simulink library "aero_sim_lib"  (Simulink 7.1)
undefined symbols (not defined in the file or in its folder): DiscIntNeverNeededParam, M, T0, tau_motor, ToverTh, Vb0, W0, X0
libraries: aero_sim_lib x24, simulink x16
(part 1 of 2)
settings Model: Creator=Administrator  LastModifiedBy=nkottens

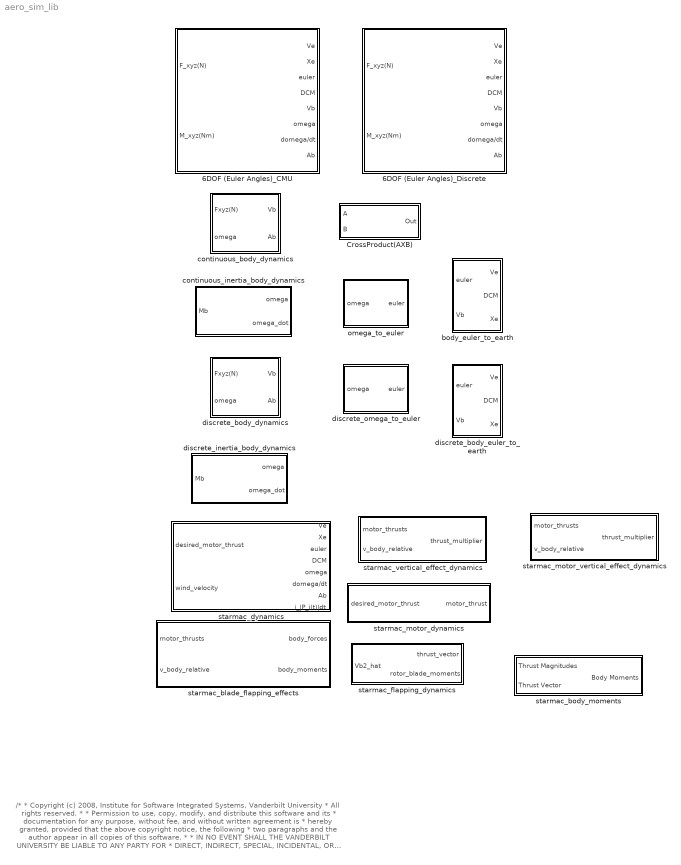
== system aero_sim_lib ==
  note: /*
      |  * Copyright (c) 2008, Institute for Software Integrated Systems, Vanderbilt University
      |  * All rights reserved.
      |  *
      |  * Permission to use, copy, modify, and distribute this software and its
      |  * documentation for any purpose, without fee, and without written agreement is
      |  * hereby granted, provided that the above copyright notice, the following
      |  * two paragraphs and the author appear in all copies of this software.
      |  *
      |  * IN NO EVENT SHALL THE VANDERBILT UNIVERSITY BE LIABLE TO ANY PARTY FOR
      |  * DIRECT, INDIRECT, SPECIAL, INCIDENTAL, OR CONSEQUENTIAL DAMAGES ARISING OUT
      |  * OF THE USE OF THIS SOFTWARE AND ITS DOCUMENTATION, EVEN IF THE VANDERBILT
      |  * UNIVERSITY HAS BEEN ADVISED OF THE POSSIBILITY OF SUCH DAMAGE.
      |  *
      |  * THE VANDERBILT UNIVERSITY SPECIFICALLY DISCLAIMS ANY WARRANTIES,
      |  * INCLUDING, BUT NOT LIMITED TO, THE IMPLIED WARRANTIES OF MERCHANTABILITY
      |  * AND FITNESS FOR A PARTICULAR PURPOSE.  THE SOFTWARE PROVIDED HEREUNDER IS
      |  * ON AN "AS IS" BASIS, AND THE VANDERBILT UNIVERSITY HAS NO OBLIGATION TO
      |  * PROVIDE MAINTENANCE, SUPPORT, UPDATES, ENHANCEMENTS, OR MODIFICATIONS.
      |  *
      |  * @author Nicholas Kottenstette
      |  */
  6DOF (Euler Angles)_CMU : Subsystem  mask{XYZe_0=zeros(3,1), Vb_0=zeros(3,1), euler_0=zeros(3,1), omega_0=zeros(3,1), M=1, I=eye(3)}
      mask prompts: XYZe_0 "Initial position in inertial axes [Xe,Ye,Ze]:"; Vb_0 "Initial velocity in body axes [U,v,w]:"; euler_0 "Initial Euler orientation [roll, pitch, yaw]=[phi,theta,psi]:"; omega_0 "Initial body rotation rates [p,q,r]=omega:"; M "Initial mass:"; I "Inertial:"
  6DOF (Euler Angles)_Discrete : Subsystem  AncestorBlock=aero_sim_lib/6DOF (Euler Angles)_CMU  mask{XYZe_0=zeros(3,1), Vb_0=zeros(3,1), euler_0=zeros(3,1), omega_0=zeros(3,1), M=1, I=eye(3), T_int=1.0}
      mask prompts: XYZe_0 "Initial position in inertial axes [Xe,Ye,Ze]:"; Vb_0 "Initial velocity in body axes [U,v,w]:"; euler_0 "Initial Euler orientation [roll, pitch, yaw]=[phi,theta,psi]:"; omega_0 "Initial body rotation rates [p,q,r]=omega:"; M "Initial mass:"; I "Inertial:"; T_int "Integrator Period:"
  CrossProduct(AXB) : Subsystem
      mask Description: Out = A x B
  body_euler_to_earth : Subsystem  AncestorBlock=aero_sim_lib/6DOF (Euler Angles)_CMU/body_euler_to_earth  mask{XYZe_0=zeros(3,1)}
      mask prompts: XYZe_0 "Initial position in inertial axes [Xe,Ye,Ze]:"
  continuous_body_dynamics : Subsystem  AncestorBlock=aero_sim_lib/6DOF (Euler Angles)_CMU/continuous_body_dynamics  mask{M=1, Vb_0=zeros(3,1)}
      mask prompts: M "Initial Mass:"; Vb_0 "Initial velocity in body axes [u,v,w]:"
  continuous_inertia_body_dynamics : Subsystem  AncestorBlock=aero_sim_lib/6DOF (Euler Angles)_CMU/continuous_inertia_body_dynamics  mask{I=eye(3), omega_0=zeros(3,1)}
      mask prompts: I "Inertia:"; omega_0 "Initial body rotation rates [p,q,r]=omega:"
  discrete_body_dynamics : Subsystem  AncestorBlock=aero_sim_lib/continuous_body_dynamics  mask{M=1, Vb_0=zeros(3,1), T_int=1.0}
      mask prompts: M "Initial Mass:"; Vb_0 "Initial velocity in body axes [u,v,w]:"; T_int "Integrator Period"
  discrete_body_euler_to_earth : Subsystem  AncestorBlock=aero_sim_lib/body_euler_to_earth  mask{XYZe_0=zeros(3,1), T_int=1.0}
      mask prompts: XYZe_0 "Initial position in inertial axes [Xe,Ye,Ze]:"; T_int "Integrator Period:"
  discrete_inertia_body_dynamics : Subsystem  AncestorBlock=aero_sim_lib/continuous_inertia_body_dynamics  mask{I=eye(3), omega_0=zeros(3,1), T_int=1.0}
      mask prompts: I "Inertia:"; omega_0 "Initial body rotation rates [p,q,r]=omega:"; T_int "Integrator Period:"
  discrete_omega_to_euler : Subsystem  AncestorBlock=aero_sim_lib/omega_to_euler  mask{euler_0=zeros(3,1), T_int=1.0}
      mask prompts: euler_0 "Initial Euler orientation [roll,pitch,yaw]:"; T_int "Integrator Period:"
  omega_to_euler : Subsystem  AncestorBlock=aero_sim_lib/6DOF (Euler Angles)_CMU/omega_to_euler  mask{euler_0=zeros(3,1)}
      mask prompts: euler_0 "Initial Euler orientation [roll,pitch,yaw]:"
  starmac_blade_flapping_effects : Subsystem  AncestorBlock=aero_sim_lib/starmac_dynamics/starmac_blade_flapping_effects
  starmac_body_moments : Subsystem  mask{dx=.3048, dz=.07, K_torque=.47}
  starmac_dynamics : Subsystem
  starmac_flapping_dynamics : Subsystem  mask{K_a1s=.009, K_beta=.23}
  starmac_motor_dynamics : Subsystem  AncestorBlock=aero_sim_lib/starmac_dynamics/starmac_motor_dynamics  mask{tau_motor=tau_motor, T_nom=M*9.8/4, thrust_max=9.8, thrust_min=0, motor_lag_enable=on, motor_variance=.01*(.05*9.8/4)^2, Ts=1/76}
      mask prompts: tau_motor "tau_motor (seconds):"; T_nom "nominal thrust (N):"; thrust_max "maximum thrust (N):"; thrust_min "minimum thrust (N):"; motor_lag_enable "Motor Lag Enabled:"; motor_variance "Motor Variance [motor_variance]:"; Ts "Motor Update Rate (seconds):"
  starmac_motor_vertical_effect_dynamics : Subsystem  mask{tau_motor=tau_motor, R=0.127, Alpha=(pi/180)*[-85:5:85], Vinf=[0:0.5:6], Vh=sqrt(9.8*[0.3:0.02:0.8]/(2*1.2*pi*.127^2)), ToverTh=ones(35,13,26)}
      mask prompts: tau_motor "motor time constant (s)"; R "radius of propeller (m)"; Alpha "Alpha (radians):"; Vinf "Vinf (m/s):"; Vh "Vh (m/s):"
      mask init:
      | rho=1.2;    % kg/m^3, density of air
      | A = pi*R^2; % m^2, area swept out by 1 rotor
  starmac_vertical_effect_dynamics : Subsystem  mask{tau_motor=tau_motor, R=0.127, Alpha=(pi/180)*[-85:5:85], Vinf=[0:0.5:6], Thrust=9.8*[0.3:0.02:0.8]}
      mask prompts: tau_motor "motor time constant (s)"; R "radius of propeller (m)"; Alpha "Alpha (radians)"; Vinf "Vinf (radians)"; Thrust "Propeller Thrust (N)"
      mask init:
      | rho = 1.2;
      | A = pi*R^2;
      | Vh = sqrt(Thrust/(2*rho*A));
      | for i = 1:length(Vh)
      |     for j = 1:length(Vinf)
      |         for k = 1:length(Alpha)
      |             Vi(k,j,i) = find_vi(Vh(i),Vinf(j),Alpha(k));
      |             ToverTh(k,j,i) = min(10,max(0.1,Vh(i)/(Vi(k,j,i)+Vinf(j)*sin(Alpha(k)))));
      |         end
      |     end
      | end

== system aero_sim_lib/6DOF (Euler Angles)_CMU ==
  note: 6 DOF System Model
  note: This subsystem models a 6 degree of freedom (6DOF) system in Euler angles.
      | A Direct Cosine Matrix (DCM) is produced to allow for easy transformations to
      | and from the reference frame of the body.  Enter appropriate Parameters in the dialog menu.
      | Follows Euler Angle Sequence (1,2,3), see Section 5.6, Representing Attitude: Euler Angles, Unit
      | Quaternions, and Rotation by James Diebel.  Interface matches that from the Aerospace Toolbox
      | for non variable mass (6DoF EoM (Body Axis) for Euler Angles).
      |
      | J. Kapinski
      | Carnegia Mellon University
      | 7/2007
      | Revised:
      | Nicholas Kottenstette, ISIS, 8/2008
  F_xyz(N) : Inport  OutDataType=sfix(16)  OutScaling=2^0
  M_xyz(Nm) : Inport  Port=2  PortDimensions=3  OutDataType=sfix(16)  OutScaling=2^0
  body_euler_to_earth : aero_sim_lib/body_euler_to_earth  SystemSampleTime=-1  XYZe_0=XYZe_0
  continuous_body_dynamics : aero_sim_lib/continuous_body_dynamics  SystemSampleTime=-1  M=M  Vb_0=Vb_0
  continuous_inertia_body_dynamics : aero_sim_lib/continuous_inertia_body_dynamics  SystemSampleTime=-1  I=I  omega_0=omega_0
  omega_to_euler : aero_sim_lib/omega_to_euler  SystemSampleTime=-1  euler_0=euler_0
  Ve : Outport  OutDataType=sfix(16)  OutScaling=2^0
  Xe : Outport  Port=2  OutDataType=sfix(16)  OutScaling=2^0
  euler : Outport  Port=3  OutDataType=sfix(16)  OutScaling=2^0
  DCM : Outport  Port=4  OutDataType=sfix(16)  OutScaling=2^0
  Vb : Outport  Port=5  OutDataType=sfix(16)  OutScaling=2^0
  omega : Outport  Port=6  OutDataType=sfix(16)  OutScaling=2^0
  domega/dt : Outport  Port=7  OutDataType=sfix(16)  OutScaling=2^0
  Ab : Outport  Port=8  OutDataType=sfix(16)  OutScaling=2^0
  wires:
  M_xyz(Nm)/1 -> continuous_inertia_body_dynamics/1
  F_xyz(N)/1 -> continuous_body_dynamics/1
  continuous_inertia_body_dynamics/1 -> omega/1, continuous_body_dynamics/2, omega_to_euler/1
  continuous_body_dynamics/1 -> Vb/1, body_euler_to_earth/2
  continuous_body_dynamics/2 -> Ab/1
  continuous_inertia_body_dynamics/2 -> domega/dt/1
  omega_to_euler/1 -> euler/1, body_euler_to_earth/1
  body_euler_to_earth/1 -> Ve/1
  body_euler_to_earth/2 -> DCM/1
  body_euler_to_earth/3 -> Xe/1

== system aero_sim_lib/6DOF (Euler Angles)_Discrete ==
  note: This subsystem models a 6 degree of freedom (6DOF) system in Euler angles.
      | A Direct Cosine Matrix (DCM) is produced to allow for easy transformations to
      | and from the reference frame of the body.  Enter appropriate Parameters in the dialog menu.
      | Follows Euler Angle Sequence (1,2,3), see Section 5.6, Representing Attitude: Euler Angles, Unit
      | Quaternions, and Rotation by James Diebel.  Interface matches that from the Aerospace Toolbox
      | for non variable mass (6DoF EoM (Body Axis) for Euler Angles).
      |
      | J. Kapinski
      | Carnegia Mellon University
      | 7/2007
      | Revised:
      | Nicholas Kottenstette, ISIS, 8/2008
  note: 6 DOF System Model
  F_xyz(N) : Inport
  M_xyz(Nm) : Inport  Port=2  PortDimensions=3
  discrete_body_dynamics : aero_sim_lib/discrete_body_dynamics  SystemSampleTime=-1  M=M  Vb_0=Vb_0  T_int=T_int
  discrete_body_euler_to_earth : aero_sim_lib/discrete_body_euler_to_earth  SystemSampleTime=-1  XYZe_0=XYZe_0  T_int=T_int
  discrete_inertia_body_dynamics : aero_sim_lib/discrete_inertia_body_dynamics  SystemSampleTime=-1  I=I  omega_0=omega_0  T_int=T_int
  discrete_omega_to_euler : aero_sim_lib/discrete_omega_to_euler  SystemSampleTime=-1  euler_0=euler_0  T_int=T_int
  Ve : Outport
  Xe : Outport  Port=2
  euler : Outport  Port=3
  DCM : Outport  Port=4
  Vb : Outport  Port=5
  omega : Outport  Port=6
  domega/dt : Outport  Port=7
  Ab : Outport  Port=8
  wires:
  discrete_body_dynamics/2 -> Ab/1
  discrete_body_dynamics/1 -> Vb/1, discrete_body_euler_to_earth/2
  F_xyz(N)/1 -> discrete_body_dynamics/1
  discrete_omega_to_euler/1 -> euler/1, discrete_body_euler_to_earth/1
  discrete_body_euler_to_earth/1 -> Ve/1
  discrete_body_euler_to_earth/2 -> DCM/1
  discrete_body_euler_to_earth/3 -> Xe/1
  M_xyz(Nm)/1 -> discrete_inertia_body_dynamics/1
  discrete_inertia_body_dynamics/1 -> omega/1, discrete_omega_to_euler/1, discrete_body_dynamics/2
  discrete_inertia_body_dynamics/2 -> domega/dt/1

== system aero_sim_lib/CrossProduct(AXB) ==
  A : Inport  OutDataType=sfix(16)  OutScaling=2^0
  B : Inport  Port=2  OutDataType=sfix(16)  OutScaling=2^0
  Fcn : Fcn  Expr=u[2]*u[6]-u[3]*u[5]
  Fcn1 : Fcn  Expr=u[3]*u[4]-u[1]*u[6]
  Fcn2 : Fcn  Expr=u[1]*u[5]-u[2]*u[4]
  Mux : Mux  Inputs=2
  Mux1 : Mux  Inputs=3
  Out : Outport  OutDataType=sfix(16)  OutScaling=2^0
  wires:
  Mux1/1 -> Out/1
  Fcn2/1 -> Mux1/3
  Fcn1/1 -> Mux1/2
  Fcn/1 -> Mux1/1
  Mux/1 -> Fcn2/1, Fcn1/1, Fcn/1
  B/1 -> Mux/2
  A/1 -> Mux/1

== system aero_sim_lib/body_euler_to_earth ==
  euler : Inport  OutDataType=sfix(16)  OutScaling=2^0
  Vb : Inport  Port=2  OutDataType=sfix(16)  OutScaling=2^0
  Constant : Constant  Value=XYZe_0  OutDataType=sfix(16)  OutScaling=2^0
  Create_DCM : Subsystem
  Math Function : Math  Operator=transpose  OutDataType=sfix(16)  OutScaling=2^0  SaturateOnIntegerOverflow=on
  Position : Integrator  InitialConditionSource=external  InitialCondition=X0
  Product2 : Product  Multiplication=Matrix(*)  OutDataType=sfix(16)  OutScaling=2^0  RndMeth=Zero
  Ve : Outport  OutDataType=sfix(16)  OutScaling=2^0
  DCM : Outport  Port=2  OutDataType=sfix(16)  OutScaling=2^0
  Xe : Outport  Port=3  OutDataType=sfix(16)  OutScaling=2^0
  wires:
  Vb/1 -> Product2/2
  euler/1 -> Create_DCM/1(euler)
  Create_DCM/1(DCM) -> Math Function/1, DCM/1
  Math Function/1 -> Product2/1
  Product2/1 -> Position/1, Ve/1
  Position/1 -> Xe/1
  Constant/1 -> Position/2

== system aero_sim_lib/continuous_body_dynamics ==
  note: Vb_dot
  Fxyz(N) : Inport  OutDataType=sfix(16)  OutScaling=2^0
  omega : Inport  Orientation=down  Port=2  OutDataType=sfix(16)  OutScaling=2^0
  Constant : Constant  Value=Vb_0  OutDataType=sfix(16)  OutScaling=2^0
  CrossProduct(AXB) : aero_sim_lib/CrossProduct(AXB)  Orientation=left  SystemSampleTime=-1
  Gain : Gain  Gain=1/M  ParameterDataType=sfix(16)  ParameterScaling=2^0  OutDataType=sfix(16)  OutScaling=2^0
  Sum : Sum  Inputs=|+-  OutDataType=sfix(16)  OutScaling=2^0
  Velocity : Integrator  InitialConditionSource=external  InitialCondition=Vb0
  Vb : Outport  OutDataType=sfix(16)  OutScaling=2^0
  Ab : Outport  Port=2  OutDataType=sfix(16)  OutScaling=2^0
  wires:
  Constant/1 -> Velocity/2
  Fxyz(N)/1 -> Gain/1
  omega/1 -> CrossProduct(AXB)/1
  Gain/1 -> Ab/1, Sum/1
  CrossProduct(AXB)/1 -> Sum/2
  Sum/1 -> Velocity/1
  Velocity/1 -> Vb/1, CrossProduct(AXB)/2  "V"

== system aero_sim_lib/continuous_inertia_body_dynamics ==
  Mb : Inport  OutDataType=sfix(16)  OutScaling=2^0
  Constant : Constant  Value=inv(I)  OutDataType=sfix(16)  OutScaling=2^0
  Constant1 : Constant  Value=I  OutDataType=sfix(16)  OutScaling=2^0
  Constant2 : Constant  Value=omega_0  OutDataType=sfix(16)  OutScaling=2^0
  CrossProduct(AXB) : aero_sim_lib/CrossProduct(AXB)  SystemSampleTime=-1
  Product : Product  Multiplication=Matrix(*)  OutDataType=sfix(16)  OutScaling=2^0  RndMeth=Zero
  Product1 : Product  Multiplication=Matrix(*)  OutDataType=sfix(16)  OutScaling=2^0  RndMeth=Zero
  Sum1 : Sum  Inputs=|-+  OutDataType=sfix(16)  OutScaling=2^0
  integrator : Integrator  InitialConditionSource=external  InitialCondition=W0
  omega : Outport  OutDataType=sfix(16)  OutScaling=2^0
  omega_dot : Outport  Port=2  OutDataType=sfix(16)  OutScaling=2^0
  wires:
  Product1/1 -> CrossProduct(AXB)/2
  Constant1/1 -> Product1/1
  Mb/1 -> Sum1/2
  CrossProduct(AXB)/1 -> Sum1/1
  integrator/1 -> Product1/2, CrossProduct(AXB)/1, omega/1
  Sum1/1 -> Product/2
  Constant2/1 -> integrator/2
  Constant/1 -> Product/1
  Product/1 -> omega_dot/1, integrator/1

== system aero_sim_lib/discrete_body_dynamics ==
  note: Vb_dot
  Fxyz(N) : Inport
  omega : Inport  Orientation=down  Port=2
  Constant : Constant  Value=Vb_0
  CrossProduct(AXB) : aero_sim_lib/CrossProduct(AXB)  Orientation=left  SystemSampleTime=-1
  Discrete-Time Integrator : DiscreteIntegrator  IntegratorMethod=Integration: Trapezoidal  InitialConditionSource=external  SampleTime=T_int  ICPrevOutput=DiscIntNeverNeededParam  ICPrevScaledInput=DiscIntNeverNeededParam
  Gain : Gain  Gain=1/M
  Sum : Sum  Inputs=|+-
  Vb : Outport
  Ab : Outport  Port=2
  wires:
  Discrete-Time Integrator/1 -> CrossProduct(AXB)/2, Vb/1  "V"
  Sum/1 -> Discrete-Time Integrator/1
  CrossProduct(AXB)/1 -> Sum/2
  Gain/1 -> Sum/1, Ab/1
  omega/1 -> CrossProduct(AXB)/1
  Fxyz(N)/1 -> Gain/1
  Constant/1 -> Discrete-Time Integrator/2

== system aero_sim_lib/discrete_body_euler_to_earth ==
  euler : Inport
  Vb : Inport  Port=2
  Constant : Constant  Value=XYZe_0
  Create_DCM : Subsystem
  Discrete-Time Integrator : DiscreteIntegrator  IntegratorMethod=Integration: Trapezoidal  InitialConditionSource=external  SampleTime=T_int  ICPrevOutput=DiscIntNeverNeededParam  ICPrevScaledInput=DiscIntNeverNeededParam
  Math Function : Math  Operator=transpose  SaturateOnIntegerOverflow=on
  Product2 : Product  Multiplication=Matrix(*)  RndMeth=Zero
  Ve : Outport
  DCM : Outport  Port=2
  Xe : Outport  Port=3
  wires:
  Constant/1 -> Discrete-Time Integrator/2
  Discrete-Time Integrator/1 -> Xe/1
  Product2/1 -> Ve/1, Discrete-Time Integrator/1
  Math Function/1 -> Product2/1
  Create_DCM/1(DCM) -> DCM/1, Math Function/1
  euler/1 -> Create_DCM/1(euler)
  Vb/1 -> Product2/2

== system aero_sim_lib/discrete_inertia_body_dynamics ==
  Mb : Inport
  Constant : Constant  Value=inv(I)
  Constant1 : Constant  Value=I
  Constant2 : Constant  Value=omega_0
  CrossProduct(AXB) : aero_sim_lib/CrossProduct(AXB)  SystemSampleTime=-1
  Discrete-Time Integrator : DiscreteIntegrator  IntegratorMethod=Integration: Trapezoidal  InitialConditionSource=external  SampleTime=T_int  ICPrevOutput=DiscIntNeverNeededParam  ICPrevScaledInput=DiscIntNeverNeededParam
  Product : Product  Multiplication=Matrix(*)  RndMeth=Zero
  Product1 : Product  Multiplication=Matrix(*)  RndMeth=Zero
  Sum1 : Sum  Inputs=|-+
  omega : Outport
  omega_dot : Outport  Port=2
  wires:
  Product/1 -> omega_dot/1, Discrete-Time Integrator/1
  Constant/1 -> Product/1
  Constant2/1 -> Discrete-Time Integrator/2
  Sum1/1 -> Product/2
  Discrete-Time Integrator/1 -> omega/1, CrossProduct(AXB)/1, Product1/2
  CrossProduct(AXB)/1 -> Sum1/1
  Mb/1 -> Sum1/2
  Constant1/1 -> Product1/1
  Product1/1 -> CrossProduct(AXB)/2

== system aero_sim_lib/discrete_omega_to_euler ==
  omega : Inport  PortDimensions=3
  Body-based-to-ref-frame-based : Subsystem
  Constant : Constant  Value=euler_0
  Discrete-Time Integrator : DiscreteIntegrator  IntegratorMethod=Integration: Trapezoidal  InitialConditionSource=external  SampleTime=T_int  ICPrevOutput=DiscIntNeverNeededParam  ICPrevScaledInput=DiscIntNeverNeededParam
  euler : Outport
  wires:
  Body-based-to-ref-frame-based/1(deuler/dt) -> Discrete-Time Integrator/1
  Discrete-Time Integrator/1 -> Body-based-to-ref-frame-based/2(euler), euler/1
  Constant/1 -> Discrete-Time Integrator/2
  omega/1 -> Body-based-to-ref-frame-based/1(omega)

== system aero_sim_lib/omega_to_euler ==
  omega : Inport  PortDimensions=3  OutDataType=sfix(16)  OutScaling=2^0
  Body-based-to-ref-frame-based : Subsystem
  Constant : Constant  Value=euler_0  OutDataType=sfix(16)  OutScaling=2^0
  integrator : Integrator  InitialConditionSource=external  InitialCondition=T0
  euler : Outport  OutDataType=sfix(16)  OutScaling=2^0
  wires:
  omega/1 -> Body-based-to-ref-frame-based/1(omega)
  Constant/1 -> integrator/2
  integrator/1 -> euler/1, Body-based-to-ref-frame-based/2(euler)
  Body-based-to-ref-frame-based/1(deuler/dt) -> integrator/1

== system aero_sim_lib/starmac_blade_flapping_effects ==
  motor_thrusts : Inport  OutDataType=sfix(16)  OutScaling=2^0
  v_body_relative : Inport  Port=2  OutDataType=sfix(16)  OutScaling=2^0
  Pick First 2 Elements : Constant  Value=[1 0 0; 0 1 0; 0 0 0]  OutDataType=sfix(16)  OutScaling=2^0
  Product : Product  OutDataType=sfix(16)  OutScaling=2^0  RndMeth=Zero
  Product2 : Product  Multiplication=Matrix(*)  OutDataType=sfix(16)  OutScaling=2^0  RndMeth=Zero
  Product4 : Product  OutDataType=sfix(16)  OutScaling=2^0  RndMeth=Zero
  Sum : Sum  Inputs=|++  OutDataType=sfix(16)  OutScaling=2^0
  Sum of Elements : Sum  Inputs=+  OutDataType=sfix(16)  OutScaling=2^-10
  starmac_body_moments : Subsystem  AncestorBlock=aero_sim_lib/starmac_body_moments  mask{dx=.3048, dz=.07, K_torque=.47}
  starmac_flapping_dynamics : Subsystem  AncestorBlock=aero_sim_lib/starmac_flapping_dynamics  mask{K_a1s=.009, K_beta=.23}
  starmac_vertical_effect_dynamics : Subsystem  AncestorBlock=aero_sim_lib/starmac_vertical_effect_dynamics  mask{tau_motor=0.1, R=0.127, Alpha=(pi/180)*[-85:5:85], Vinf=[0:0.5:6], Thrust=9.8*[0.3:0.02:0.8]}
      mask prompts: tau_motor "motor time constant (s)"; R "radius of propeller (m)"; Alpha "Alpha (radians)"; Vinf "Vinf (radians)"; Thrust "Propeller Thrust (N)"
      mask init: same as aero_sim_lib/starmac_vertical_effect_dynamics
  body_forces : Outport  OutDataType=sfix(16)  OutScaling=2^0
  body_moments : Outport  Port=2  OutDataType=sfix(16)  OutScaling=2^0
  wires:
  Product/1 -> starmac_body_moments/1(Thrust Magnitudes), Sum of Elements/1
  starmac_vertical_effect_dynamics/1(thrust_multiplier) -> Product/2
  motor_thrusts/1 -> starmac_vertical_effect_dynamics/1(motor_thrusts), Product/1
  Pick First 2 Elements/1 -> Product2/1
  v_body_relative/1 -> starmac_vertical_effect_dynamics/2(v_body_relative), Product2/2
  Product2/1 -> starmac_flapping_dynamics/1(Vb2_hat)
  Sum of Elements/1 -> Product4/1
  Product4/1 -> body_forces/1
  starmac_flapping_dynamics/1(thrust_vector) -> starmac_body_moments/2(Thrust Vector), Product4/2
  starmac_body_moments/1(Body Moments) -> Sum/1
  Sum/1 -> body_moments/1
  starmac_flapping_dynamics/2(rotor_blade_moments) -> Sum/2

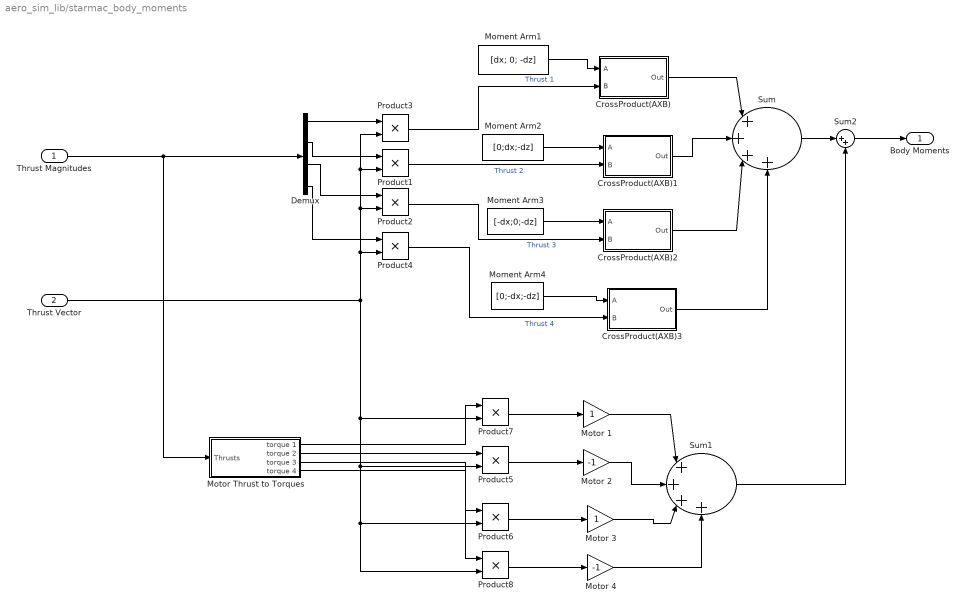
== system aero_sim_lib/starmac_body_moments ==
  Thrust Magnitudes : Inport  OutDataType=sfix(16)  OutScaling=2^0
  Thrust Vector : Inport  Port=2  OutDataType=sfix(16)  OutScaling=2^0
  CrossProduct(AXB) : Subsystem
  CrossProduct(AXB)1 : Subsystem
  CrossProduct(AXB)2 : Subsystem
  CrossProduct(AXB)3 : Subsystem
  Demux : Demux
  Moment Arm1 : Constant  Value=[dx; 0; -dz]  OutDataType=sfix(16)  OutScaling=2^0
  Moment Arm2 : Constant  Value=[0;dx;-dz]  OutDataType=sfix(16)  OutScaling=2^0
  Moment Arm3 : Constant  Value=[-dx;0;-dz]  OutDataType=sfix(16)  OutScaling=2^0
  Moment Arm4 : Constant  Value=[0;-dx;-dz]  OutDataType=sfix(16)  OutScaling=2^0
  Motor 1 : Gain  ParameterDataType=sfix(16)  ParameterScaling=2^0  OutDataType=sfix(16)  OutScaling=2^0
  Motor 2 : Gain  Gain=-1  ParameterDataType=sfix(16)  ParameterScaling=2^0  OutDataType=sfix(16)  OutScaling=2^0
  Motor 3 : Gain  ParameterDataType=sfix(16)  ParameterScaling=2^0  OutDataType=sfix(16)  OutScaling=2^0
  Motor 4 : Gain  Gain=-1  ParameterDataType=sfix(16)  ParameterScaling=2^0  OutDataType=sfix(16)  OutScaling=2^0
  Motor Thrust to Torques : Subsystem
  Product{1..8} (8 alike) : Product  OutDataType=sfix(16)  OutScaling=2^0  RndMeth=Zero
  Sum : Sum  Inputs=|++++  OutDataType=sfix(16)  OutScaling=2^0
  Sum1 : Sum  Inputs=|++++  OutDataType=sfix(16)  OutScaling=2^0
  Sum2 : Sum  Inputs=|++  OutDataType=sfix(16)  OutScaling=2^0
  Body Moments : Outport  OutDataType=sfix(16)  OutScaling=2^0
  wires:
  CrossProduct(AXB)1/1(Out) -> Sum/2
  Motor Thrust to Torques/4(torque 4) -> Product8/1
  Motor Thrust to Torques/3(torque 3) -> Product6/1
  Motor Thrust to Torques/2(torque 2) -> Product5/1
  Motor Thrust to Torques/1(torque 1) -> Product7/1
  Product8/1 -> Motor 4/1
  Product6/1 -> Motor 3/1
  Product5/1 -> Motor 2/1
  Product7/1 -> Motor 1/1
  Sum2/1 -> Body Moments/1
  Sum1/1 -> Sum2/2
  Sum/1 -> Sum2/1
  Motor 4/1 -> Sum1/4
  Motor 3/1 -> Sum1/3
  Motor 2/1 -> Sum1/2
  Motor 1/1 -> Sum1/1
  CrossProduct(AXB)3/1(Out) -> Sum/4
  CrossProduct(AXB)2/1(Out) -> Sum/3
  CrossProduct(AXB)/1(Out) -> Sum/1
  Product4/1 -> CrossProduct(AXB)3/2(B)  "Thrust 4"
  Moment Arm4/1 -> CrossProduct(AXB)3/1(A)
  Product2/1 -> CrossProduct(AXB)2/2(B)  "Thrust 3"
  Moment Arm3/1 -> CrossProduct(AXB)2/1(A)
  Product1/1 -> CrossProduct(AXB)1/2(B)  "Thrust 2"
  Moment Arm2/1 -> CrossProduct(AXB)1/1(A)
  Product3/1 -> CrossProduct(AXB)/2(B)  "Thrust 1"
  Moment Arm1/1 -> CrossProduct(AXB)/1(A)
  Thrust Vector/1 -> Product8/2, Product6/2, Product5/2, Product7/2, Product4/2, Product2/2, Product1/2, Product3/2
  Demux/4 -> Product4/1
  Demux/3 -> Product2/1
  Demux/2 -> Product1/1
  Demux/1 -> Product3/1
  Thrust Magnitudes/1 -> Motor Thrust to Torques/1(Thrusts), Demux/1

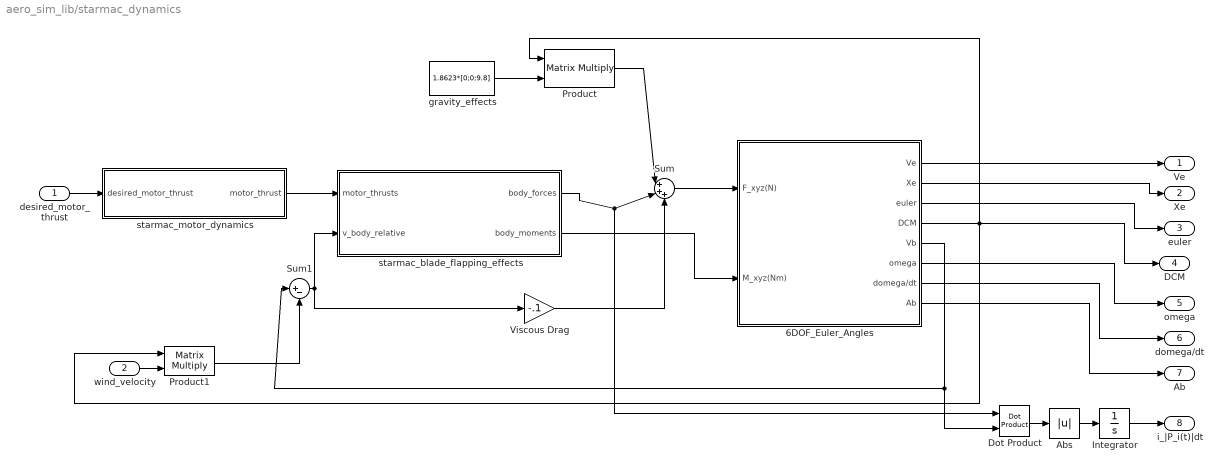
== system aero_sim_lib/starmac_dynamics ==
  desired_motor_thrust : Inport  OutDataType=sfix(16)  OutScaling=2^0
  wind_velocity : Inport  Port=2  OutDataType=sfix(16)  OutScaling=2^0
  6DOF_Euler_Angles : Subsystem  AncestorBlock=aero_sim_lib/6DOF (Euler Angles)_CMU  mask{XYZe_0=[0.1;0.2;0], Vb_0=[0;0;0], euler_0=[0;0;0], omega_0=[0;0;0], M=1.8623, I=diag([0.02759 0.02771 0.04806])}
      mask prompts: XYZe_0 "Initial position in inertial axes [Xe,Ye,Ze]:"; Vb_0 "Initial velocity in body axes [U,v,w]:"; euler_0 "Initial Euler orientation [roll, pitch, yaw]=[phi,theta,psi]:"; omega_0 "Initial body rotation rates [p,q,r]=omega:"; M "Initial mass:"; I "Inertial:"
  Abs : Abs  OutDataType=sfix(16)  OutScaling=2^0
  Dot Product : simulink/Math Operations/Dot Product  InputSameDT=on  OutDataType=sfix(16)  OutScaling=2^-10  DoSatur=off
  Integrator : Integrator
  Product : Product  Multiplication=Matrix(*)  OutDataType=sfix(16)  OutScaling=2^0  RndMeth=Zero
  Product1 : Product  Multiplication=Matrix(*)  OutDataType=sfix(16)  OutScaling=2^0  RndMeth=Zero
  Sum : Sum  Inputs=|+++  OutDataType=sfix(16)  OutScaling=2^0
  Sum1 : Sum  Inputs=|+-  OutDataType=sfix(16)  OutScaling=2^0
  Viscous Drag : Gain  Gain=-.1  ParameterDataType=sfix(16)  ParameterScaling=2^0  OutDataType=sfix(16)  OutScaling=2^0
  gravity_effects : Constant  Value=1.8623*[0;0;9.8]  OutDataType=sfix(16)  OutScaling=2^0
  starmac_blade_flapping_effects : Subsystem  AncestorBlock=aero_sim_lib/starmac_blade_flapping_effects
  starmac_motor_dynamics : Subsystem  AncestorBlock=aero_sim_lib/starmac_motor_dynamics  mask{tau_motor=.1, T_nom=1.8263*9.8/4, thrust_max=9.8, thrust_min=0, motor_lag_enable=on, motor_variance=.01*(.05*9.8/4)^2, Ts=1/76}
      mask prompts: tau_motor "tau_motor (seconds):"; T_nom "nominal thrust (N):"; thrust_max "maximum thrust (N):"; thrust_min "minimum thrust (N):"; motor_lag_enable "Motor Lag Enabled:"; motor_variance "Motor Variance [motor_variance]:"; Ts "Motor Update Rate (seconds):"
  Ve : Outport  OutDataType=sfix(16)  OutScaling=2^0
  Xe : Outport  Port=2  OutDataType=sfix(16)  OutScaling=2^0
  euler : Outport  Port=3  OutDataType=sfix(16)  OutScaling=2^0
  DCM : Outport  Port=4  OutDataType=sfix(16)  OutScaling=2^0
  omega : Outport  Port=5  OutDataType=sfix(16)  OutScaling=2^0
  domega/dt : Outport  Port=6  OutDataType=sfix(16)  OutScaling=2^0
  Ab : Outport  Port=7  OutDataType=sfix(16)  OutScaling=2^0
  i_|P_i(t)|dt : Outport  Port=8  OutDataType=sfix(16)  OutScaling=2^0
  wires:
  wind_velocity/1 -> Product1/2
  desired_motor_thrust/1 -> starmac_motor_dynamics/1(desired_motor_thrust)
  starmac_blade_flapping_effects/1(body_forces) -> Sum/2, Dot Product/1
  starmac_blade_flapping_effects/2(body_moments) -> 6DOF_Euler_Angles/2(M_xyz(Nm))
  Viscous Drag/1 -> Sum/3
  6DOF_Euler_Angles/5(Vb) -> Sum1/1, Dot Product/2
  Product1/1 -> Sum1/2
  Sum1/1 -> Viscous Drag/1, starmac_blade_flapping_effects/2(v_body_relative)
  gravity_effects/1 -> Product/2
  6DOF_Euler_Angles/4(DCM) -> Product1/1, Product/1, DCM/1
  Sum/1 -> 6DOF_Euler_Angles/1(F_xyz(N))
  Product/1 -> Sum/1
  starmac_motor_dynamics/1(motor_thrust) -> starmac_blade_flapping_effects/1(motor_thrusts)
  6DOF_Euler_Angles/1(Ve) -> Ve/1
  6DOF_Euler_Angles/2(Xe) -> Xe/1
  6DOF_Euler_Angles/3(euler) -> euler/1
  6DOF_Euler_Angles/6(omega) -> omega/1
  6DOF_Euler_Angles/7(domega/dt) -> domega/dt/1
  6DOF_Euler_Angles/8(Ab) -> Ab/1
  Integrator/1 -> i_|P_i(t)|dt/1
  Dot Product/1 -> Abs/1
  Abs/1 -> Integrator/1

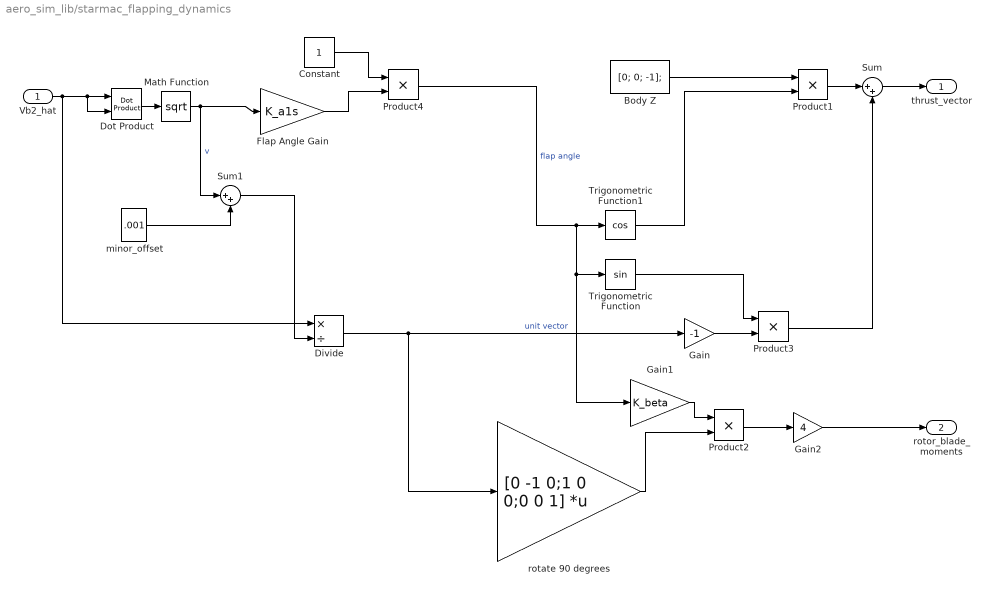
== system aero_sim_lib/starmac_flapping_dynamics ==
  Vb2_hat : Inport  OutDataType=sfix(16)  OutScaling=2^0
  "Body Z " : Constant  Value=[0; 0; -1];  OutDataType=sfix(16)  OutScaling=2^0
  Constant : Constant  OutDataType=sfix(16)  OutScaling=2^0
  Divide : Product  Inputs=*/  OutDataType=sfix(16)  OutScaling=2^-10
  Dot Product : simulink/Math Operations/Dot Product  InputSameDT=on  OutDataType=sfix(16)  OutScaling=2^-10  DoSatur=off
  Flap Angle Gain : Gain  Gain=K_a1s  ParameterDataType=sfix(16)  ParameterScaling=2^0  OutDataType=sfix(16)  OutScaling=2^0
  Gain : Gain  Gain=-1  ParameterDataType=sfix(16)  ParameterScaling=2^0  OutDataType=sfix(16)  OutScaling=2^0
  Gain1 : Gain  Gain=K_beta  ParameterDataType=sfix(16)  ParameterScaling=2^0  OutDataType=sfix(16)  OutScaling=2^0
  Gain2 : Gain  Gain=4  ParameterDataType=sfix(16)  ParameterScaling=2^0  OutDataType=sfix(16)  OutScaling=2^0
  Math Function : Math  Operator=sqrt  OutDataType=sfix(16)  OutScaling=2^0  SaturateOnIntegerOverflow=on
  Product{1..4} (4 alike) : Product  OutDataType=sfix(16)  OutScaling=2^0  RndMeth=Zero
  Sum : Sum  Inputs=|++  OutDataType=sfix(16)  OutScaling=2^0
  Sum1 : Sum  Inputs=|++  OutDataType=sfix(16)  OutScaling=2^0
  Trigonometric Function : Trigonometry
  Trigonometric Function1 : Trigonometry  Operator=cos
  minor_offset : Constant  Value=.001  OutDataType=sfix(16)  OutScaling=2^0
  rotate 90 degrees : Gain  Gain=[0 -1 0;1 0 0;0 0 1]  Multiplication=Matrix(K*u)  ParameterDataType=sfix(16)  ParameterScaling=2^0  OutDataType=sfix(16)  OutScaling=2^0
  thrust_vector : Outport  OutDataType=sfix(16)  OutScaling=2^0
  rotor_blade_moments : Outport  Port=2  OutDataType=sfix(16)  OutScaling=2^0
  wires:
  minor_offset/1 -> Sum1/2
  Sum1/1 -> Divide/2
  Divide/1 -> rotate 90 degrees/1, Gain/1  "unit vector"
  Product4/1 -> Trigonometric Function1/1, Trigonometric Function/1, Gain1/1  "flap angle"
  Vb2_hat/1 -> Divide/1, Dot Product/1, Dot Product/2
  Dot Product/1 -> Math Function/1
  Math Function/1 -> Sum1/1, Flap Angle Gain/1  "v"
  Trigonometric Function1/1 -> Product1/2
  Trigonometric Function/1 -> Product3/1
  Product3/1 -> Sum/2
  Gain/1 -> Product3/2
  Product1/1 -> Sum/1
  "Body Z "/1 -> Product1/1
  Sum/1 -> thrust_vector/1
  Gain2/1 -> rotor_blade_moments/1
  Product2/1 -> Gain2/1
  rotate 90 degrees/1 -> Product2/2
  Gain1/1 -> Product2/1
  Flap Angle Gain/1 -> Product4/2
  Constant/1 -> Product4/1

== system aero_sim_lib/starmac_motor_dynamics ==
  desired_motor_thrust : Inport  OutDataType=sfix(16)  OutScaling=2^0
  Band-Limited White Noise : simulink/Sources/Band-Limited White Noise  SystemSampleTime=-1  Cov=Ts*motor_variance*ones(4,1)  Ts=Ts  seed=22341+[0 1 2 3]'
  Constant : Constant  Value=motor_lag_enable  OutDataType=sfix(16)  OutScaling=2^0
  Saturation : Saturate  UpperLimit=thrust_max*ones(4,1)  LowerLimit=thrust_min*ones(4,1)
  State-Space : StateSpace  A=-(1/tau_motor)*eye(4)  B=(1/tau_motor)*eye(4)  C=eye(4)  D=zeros(4,4)  X0=T_nom*ones(4,1)
  Sum : Sum  Inputs=|++  OutDataType=sfix(16)  OutScaling=2^0
  Switch : Switch  Criteria=u2 > Threshold  OutDataType=sfix(16)  OutScaling=2^0
  motor_thrust : Outport  OutDataType=sfix(16)  OutScaling=2^0
  wires:
  Constant/1 -> Switch/2
  Switch/1 -> Saturation/1
  State-Space/1 -> Switch/1
  Band-Limited White Noise/1 -> Sum/2
  Saturation/1 -> Sum/1
  Sum/1 -> motor_thrust/1
  desired_motor_thrust/1 -> Switch/3, State-Space/1

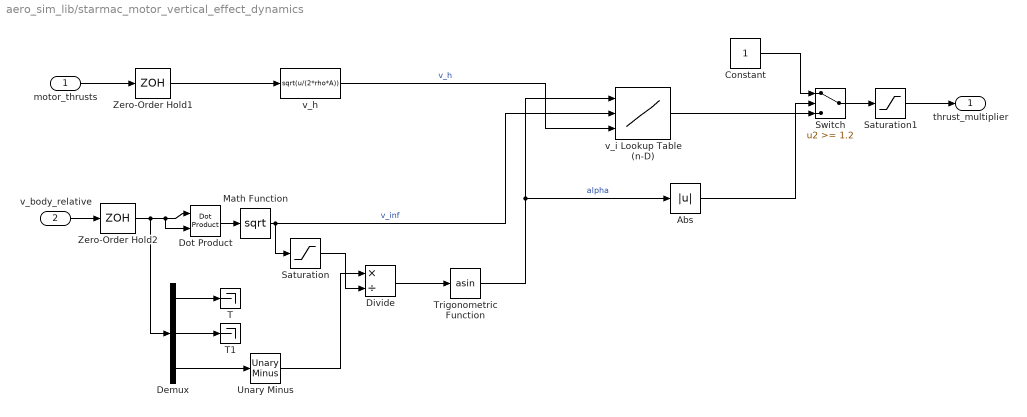
== system aero_sim_lib/starmac_motor_vertical_effect_dynamics ==
  motor_thrusts : Inport  OutDataType=sfix(16)  OutScaling=2^0
  v_body_relative : Inport  Port=2  OutDataType=sfix(16)  OutScaling=2^0
  Abs : Abs
  Constant : Constant  OutDataType=sfix(16)  OutScaling=2^0
  Demux : Demux  Outputs=3
  Divide : Product  Inputs=*/  OutDataType=sfix(16)  OutScaling=2^-10
  Dot Product : simulink/Math Operations/Dot Product  InputSameDT=on  OutDataType=sfix(16)  OutScaling=2^-10  DoSatur=off
  Math Function : Math  Operator=sqrt  OutDataType=sfix(16)  OutScaling=2^0  SaturateOnIntegerOverflow=on
  Saturation : Saturate  UpperLimit=500000  LowerLimit=0.0000000001
  Saturation1 : Saturate  UpperLimit=2  LowerLimit=0.5
  Switch : Switch  Threshold=1.2
  T : Terminator
  T1 : Terminator
  Trigonometric Function : Trigonometry  Operator=asin
  Unary Minus : simulink/Math Operations/Unary Minus  DoSatur=off
  Zero-Order Hold1 : ZeroOrderHold  SampleTime=tau_motor
  Zero-Order Hold2 : ZeroOrderHold  SampleTime=tau_motor
  "v_h " : Fcn  Expr=sqrt(u/(2*rho*A))
  v_i Lookup Table (n-D) : Lookup_n-D  NumberOfTableDimensions=3  BreakpointsForDimension1=Alpha  BreakpointsForDimension2=Vinf  BreakpointsForDimension3=Vh  BeginIndexSearchUsingPreviousIndexResult=on  Table=ToverTh  InterpMethod=Cubic spline  InputSameDT=on
  thrust_multiplier : Outport  OutDataType=sfix(16)  OutScaling=2^0
  wires:
  "v_h "/1 -> v_i Lookup Table (n-D)/3  "v_h"
  Saturation1/1 -> thrust_multiplier/1
  Zero-Order Hold2/1 -> Dot Product/1, Dot Product/2, Demux/1
  Zero-Order Hold1/1 -> "v_h "/1
  motor_thrusts/1 -> Zero-Order Hold1/1
  v_body_relative/1 -> Zero-Order Hold2/1
  Dot Product/1 -> Math Function/1
  Math Function/1 -> v_i Lookup Table (n-D)/2, Saturation/1  "v_inf"
  Demux/1 -> T/1
  Demux/2 -> T1/1
  Divide/1 -> Trigonometric Function/1
  Trigonometric Function/1 -> Abs/1, v_i Lookup Table (n-D)/1  "alpha"
  Switch/1 -> Saturation1/1
  v_i Lookup Table (n-D)/1 -> Switch/3
  Constant/1 -> Switch/1
  Abs/1 -> Switch/2
  Unary Minus/1 -> Divide/1
  Demux/3 -> Unary Minus/1
  Saturation/1 -> Divide/2

== system aero_sim_lib/starmac_vertical_effect_dynamics ==
  motor_thrusts : Inport  OutDataType=sfix(16)  OutScaling=2^0
  v_body_relative : Inport  Port=2  OutDataType=sfix(16)  OutScaling=2^0
  Demux : Demux
  Mux : Mux
  starmac_motor_vertical_effect_dynamics : Subsystem  AncestorBlock=aero_sim_lib/starmac_motor_vertical_effect_dynamics  mask{tau_motor=tau_motor, R=R, Alpha=Alpha, Vinf=Vinf, Vh=Vh, ToverTh=ToverTh}
      mask prompts: tau_motor "motor time constant (s)"; R "radius of propeller (m)"; Alpha "Alpha (radians):"; Vinf "Vinf (m/s):"; Vh "Vh (m/s):"
      mask init:
      | rho=1.2;    % kg/m^3, density of air
      | A = pi*R^2; % m^2, area swept out by 1 rotor
  starmac_motor_vertical_effect_dynamics1 : Subsystem  AncestorBlock=aero_sim_lib/starmac_motor_vertical_effect_dynamics  mask{tau_motor=tau_motor, R=R, Alpha=Alpha, Vinf=Vinf, Vh=Vh, ToverTh=ToverTh}
      mask prompts: tau_motor "motor time constant (s)"; R "radius of propeller (m)"; Alpha "Alpha (radians):"; Vinf "Vinf (m/s):"; Vh "Vh (m/s):"
      mask init:
      | rho=1.2;    % kg/m^3, density of air
      | A = pi*R^2; % m^2, area swept out by 1 rotor
  starmac_motor_vertical_effect_dynamics2 : Subsystem  AncestorBlock=aero_sim_lib/starmac_motor_vertical_effect_dynamics  mask{tau_motor=tau_motor, R=R, Alpha=Alpha, Vinf=Vinf, Vh=Vh, ToverTh=ToverTh}
      mask prompts: tau_motor "motor time constant (s)"; R "radius of propeller (m)"; Alpha "Alpha (radians):"; Vinf "Vinf (m/s):"; Vh "Vh (m/s):"
      mask init:
      | rho=1.2;    % kg/m^3, density of air
      | A = pi*R^2; % m^2, area swept out by 1 rotor
  starmac_motor_vertical_effect_dynamics3 : Subsystem  AncestorBlock=aero_sim_lib/starmac_motor_vertical_effect_dynamics  mask{tau_motor=tau_motor, R=R, Alpha=Alpha, Vinf=Vinf, Vh=Vh, ToverTh=ToverTh}
      mask prompts: tau_motor "motor time constant (s)"; R "radius of propeller (m)"; Alpha "Alpha (radians):"; Vinf "Vinf (m/s):"; Vh "Vh (m/s):"
      mask init:
      | rho=1.2;    % kg/m^3, density of air
      | A = pi*R^2; % m^2, area swept out by 1 rotor
  thrust_multiplier : Outport  OutDataType=sfix(16)  OutScaling=2^0
  wires:
  motor_thrusts/1 -> Demux/1
  Mux/1 -> thrust_multiplier/1
  Demux/1 -> starmac_motor_vertical_effect_dynamics/1(motor_thrusts)
  Demux/2 -> starmac_motor_vertical_effect_dynamics1/1(motor_thrusts)
  Demux/3 -> starmac_motor_vertical_effect_dynamics2/1(motor_thrusts)
  Demux/4 -> starmac_motor_vertical_effect_dynamics3/1(motor_thrusts)
  starmac_motor_vertical_effect_dynamics/1(thrust_multiplier) -> Mux/1
  starmac_motor_vertical_effect_dynamics1/1(thrust_multiplier) -> Mux/2
  starmac_motor_vertical_effect_dynamics2/1(thrust_multiplier) -> Mux/3
  starmac_motor_vertical_effect_dynamics3/1(thrust_multiplier) -> Mux/4
  v_body_relative/1 -> starmac_motor_vertical_effect_dynamics2/2(v_body_relative), starmac_motor_vertical_effect_dynamics3/2(v_body_relative), starmac_motor_vertical_effect_dynamics1/2(v_body_relative), starmac_motor_vertical_effect_dynamics/2(v_body_relative)

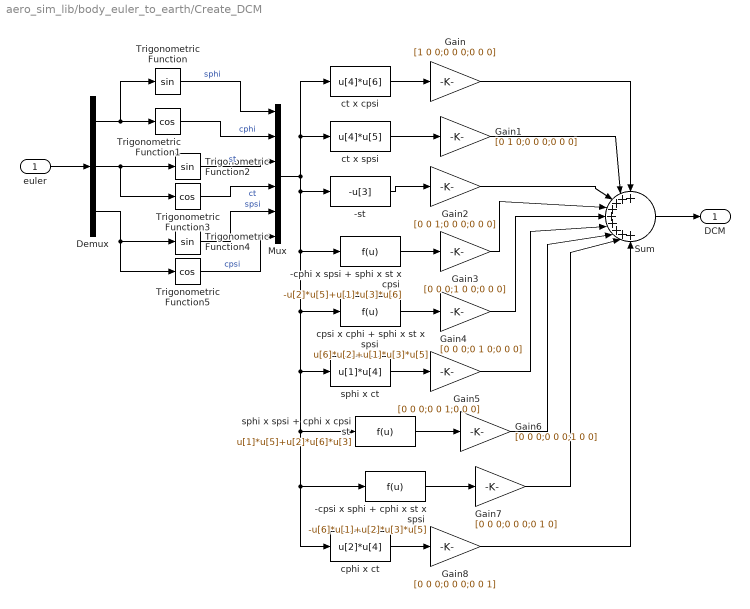
== system aero_sim_lib/body_euler_to_earth/Create_DCM ==
  euler : Inport  OutDataType=sfix(16)  OutScaling=2^0
  -cphi x spsi + sphi x st x cpsi : Fcn  Expr=-u[2]*u[5]+u[1]*u[3]*u[6]
  -cpsi x sphi + cphi x st x spsi : Fcn  Expr=-u[6]*u[1]+u[2]*u[3]*u[5]
  -st : Fcn  Expr=-u[3]
  Demux : Demux  Outputs=3
  Gain : Gain  Gain=[1 0 0;0 0 0;0 0 0]  ParameterDataType=sfix(16)  ParameterScaling=2^0  OutDataType=sfix(16)  OutScaling=2^0
  Gain1 : Gain  Gain=[0 1 0;0 0 0;0 0 0]  ParameterDataType=sfix(16)  ParameterScaling=2^0  OutDataType=sfix(16)  OutScaling=2^0
  Gain2 : Gain  Gain=[0 0 1;0 0 0;0 0 0]  ParameterDataType=sfix(16)  ParameterScaling=2^0  OutDataType=sfix(16)  OutScaling=2^0
  Gain3 : Gain  Gain=[0 0 0;1 0 0;0 0 0]  ParameterDataType=sfix(16)  ParameterScaling=2^0  OutDataType=sfix(16)  OutScaling=2^0
  Gain4 : Gain  Gain=[0 0 0;0 1 0;0 0 0]  ParameterDataType=sfix(16)  ParameterScaling=2^0  OutDataType=sfix(16)  OutScaling=2^0
  Gain5 : Gain  Gain=[0 0 0;0 0 1;0 0 0]  ParameterDataType=sfix(16)  ParameterScaling=2^0  OutDataType=sfix(16)  OutScaling=2^0
  Gain6 : Gain  Gain=[0 0 0;0 0 0;1 0 0]  ParameterDataType=sfix(16)  ParameterScaling=2^0  OutDataType=sfix(16)  OutScaling=2^0
  Gain7 : Gain  Gain=[0 0 0;0 0 0;0 1 0]  ParameterDataType=sfix(16)  ParameterScaling=2^0  OutDataType=sfix(16)  OutScaling=2^0
  Gain8 : Gain  Gain=[0 0 0;0 0 0;0 0 1]  ParameterDataType=sfix(16)  ParameterScaling=2^0  OutDataType=sfix(16)  OutScaling=2^0
  Mux : Mux  Inputs=6
  Sum : Sum  Inputs=+++++++++  OutDataType=sfix(16)  OutScaling=2^0
  Trigonometric Function : Trigonometry
  Trigonometric Function1 : Trigonometry  Operator=cos
  Trigonometric Function2 : Trigonometry
  Trigonometric Function3 : Trigonometry  Operator=cos
  Trigonometric Function4 : Trigonometry
  Trigonometric Function5 : Trigonometry  Operator=cos
  cphi x ct : Fcn  Expr=u[2]*u[4]
  cpsi x cphi + sphi x st x spsi : Fcn  Expr=u[6]*u[2]+u[1]*u[3]*u[5]
  ct x cpsi : Fcn  Expr=u[4]*u[6]
  ct x spsi : Fcn  Expr=u[4]*u[5]
  sphi x ct : Fcn  Expr=u[1]*u[4]
  sphi x spsi + cphi x cpsi st : Fcn  Expr=u[1]*u[5]+u[2]*u[6]*u[3]
  DCM : Outport  OutDataType=sfix(16)  OutScaling=2^0
  wires:
  Trigonometric Function/1 -> Mux/1  "sphi"
  Trigonometric Function3/1 -> Mux/4  "ct"
  Trigonometric Function4/1 -> Mux/5  "spsi"
  Trigonometric Function5/1 -> Mux/6  "cpsi"
  euler/1 -> Demux/1
  Demux/1 -> Trigonometric Function/1, Trigonometric Function1/1
  Demux/2 -> Trigonometric Function2/1, Trigonometric Function3/1
  Demux/3 -> Trigonometric Function4/1, Trigonometric Function5/1
  Trigonometric Function1/1 -> Mux/2  "cphi"
  Trigonometric Function2/1 -> Mux/3  "st"
  Mux/1 -> ct x cpsi/1, ct x spsi/1, -st/1, -cphi x spsi + sphi x st x cpsi/1, cpsi x cphi + sphi x st x spsi/1, sphi x ct/1, sphi x spsi + cphi x cpsi st/1, -cpsi x sphi + cphi x st x spsi/1, cphi x ct/1
  ct x cpsi/1 -> Gain/1
  Gain/1 -> Sum/1
  ct x spsi/1 -> Gain1/1
  Gain1/1 -> Sum/2
  -st/1 -> Gain2/1
  Gain2/1 -> Sum/3
  -cphi x spsi + sphi x st x cpsi/1 -> Gain3/1
  Gain3/1 -> Sum/4
  cpsi x cphi + sphi x st x spsi/1 -> Gain4/1
  Gain4/1 -> Sum/5
  sphi x ct/1 -> Gain5/1
  Gain5/1 -> Sum/6
  sphi x spsi + cphi x cpsi st/1 -> Gain6/1
  Gain6/1 -> Sum/7
  -cpsi x sphi + cphi x st x spsi/1 -> Gain7/1
  Gain7/1 -> Sum/8
  cphi x ct/1 -> Gain8/1
  Gain8/1 -> Sum/9
  Sum/1 -> DCM/1

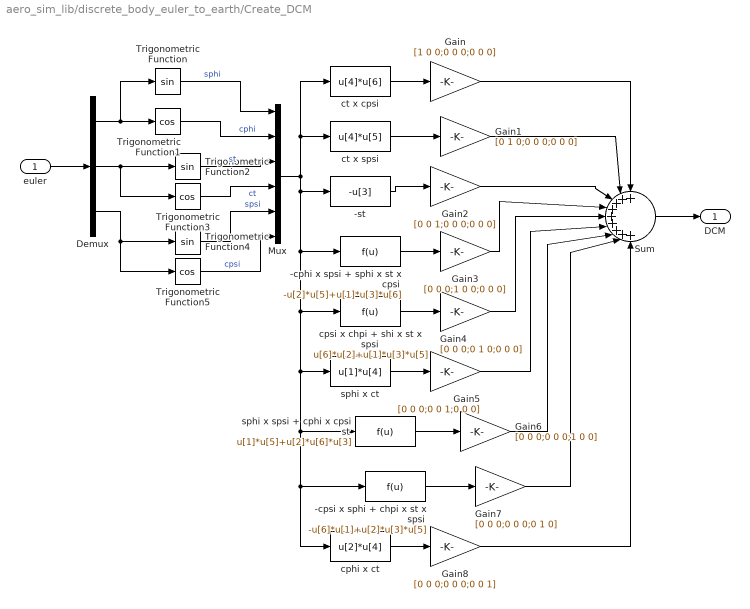
== system aero_sim_lib/discrete_body_euler_to_earth/Create_DCM ==
  euler : Inport
  -cphi x spsi + sphi x st x cpsi : Fcn  Expr=-u[2]*u[5]+u[1]*u[3]*u[6]
  -cpsi x sphi + chpi x st x spsi : Fcn  Expr=-u[6]*u[1]+u[2]*u[3]*u[5]
  -st : Fcn  Expr=-u[3]
  Demux : Demux  Outputs=3
  Gain : Gain  Gain=[1 0 0;0 0 0;0 0 0]
  Gain1 : Gain  Gain=[0 1 0;0 0 0;0 0 0]
  Gain2 : Gain  Gain=[0 0 1;0 0 0;0 0 0]
  Gain3 : Gain  Gain=[0 0 0;1 0 0;0 0 0]
  Gain4 : Gain  Gain=[0 0 0;0 1 0;0 0 0]
  Gain5 : Gain  Gain=[0 0 0;0 0 1;0 0 0]
  Gain6 : Gain  Gain=[0 0 0;0 0 0;1 0 0]
  Gain7 : Gain  Gain=[0 0 0;0 0 0;0 1 0]
  Gain8 : Gain  Gain=[0 0 0;0 0 0;0 0 1]
  Mux : Mux  Inputs=6
  Sum : Sum  Inputs=+++++++++
  Trigonometric Function : Trigonometry
  Trigonometric Function1 : Trigonometry  Operator=cos
  Trigonometric Function2 : Trigonometry
  Trigonometric Function3 : Trigonometry  Operator=cos
  Trigonometric Function4 : Trigonometry
  Trigonometric Function5 : Trigonometry  Operator=cos
  cphi x ct : Fcn  Expr=u[2]*u[4]
  cpsi x chpi + shi x st x spsi : Fcn  Expr=u[6]*u[2]+u[1]*u[3]*u[5]
  ct x cpsi : Fcn  Expr=u[4]*u[6]
  ct x spsi : Fcn  Expr=u[4]*u[5]
  sphi x ct : Fcn  Expr=u[1]*u[4]
  sphi x spsi + cphi x cpsi st : Fcn  Expr=u[1]*u[5]+u[2]*u[6]*u[3]
  DCM : Outport
  wires:
  Sum/1 -> DCM/1
  Gain8/1 -> Sum/9
  cphi x ct/1 -> Gain8/1
  Gain7/1 -> Sum/8
  -cpsi x sphi + chpi x st x spsi/1 -> Gain7/1
  Gain6/1 -> Sum/7
  sphi x spsi + cphi x cpsi st/1 -> Gain6/1
  Gain5/1 -> Sum/6
  sphi x ct/1 -> Gain5/1
  Gain4/1 -> Sum/5
  cpsi x chpi + shi x st x spsi/1 -> Gain4/1
  Gain3/1 -> Sum/4
  -cphi x spsi + sphi x st x cpsi/1 -> Gain3/1
  Gain2/1 -> Sum/3
  -st/1 -> Gain2/1
  Gain1/1 -> Sum/2
  ct x spsi/1 -> Gain1/1
  Gain/1 -> Sum/1
  ct x cpsi/1 -> Gain/1
  Mux/1 -> cphi x ct/1, -cpsi x sphi + chpi x st x spsi/1, sphi x spsi + cphi x cpsi st/1, sphi x ct/1, cpsi x chpi + shi x st x spsi/1, -cphi x spsi + sphi x st x cpsi/1, -st/1, ct x spsi/1, ct x cpsi/1
  Trigonometric Function2/1 -> Mux/3  "st"
  Trigonometric Function1/1 -> Mux/2  "cphi"
  Demux/3 -> Trigonometric Function5/1, Trigonometric Function4/1
  Demux/2 -> Trigonometric Function3/1, Trigonometric Function2/1
  Demux/1 -> Trigonometric Function1/1, Trigonometric Function/1
  euler/1 -> Demux/1
  Trigonometric Function5/1 -> Mux/6  "cpsi"
  Trigonometric Function4/1 -> Mux/5  "spsi"
  Trigonometric Function3/1 -> Mux/4  "ct"
  Trigonometric Function/1 -> Mux/1  "sphi"

== system aero_sim_lib/discrete_omega_to_euler/Body-based-to-ref-frame-based ==
  note: dF/dt = P + Q sinF tanQ + R cosF tanQ
      | dQ/dt = Q cosF - R sinF
      | dY/dt = Q sinF secQ + R cosF secQ
  omega : Inport
  euler : Inport  Port=2
  Fcn : Fcn  Expr=u[1]+u[2]*sin(u[4])*tan(u[5])+u[3]*cos(u[4])*tan(u[5])
  Fcn1 : Fcn  Expr=u[2]*cos(u[4])-u[3]*sin(u[4])
  Fcn2 : Fcn  Expr=u[2]*(sin(u[4])/cos(u[5])) + u[3]*(cos(u[4])/cos(u[5]))
  Mux : Mux  Inputs=2
  Mux1 : Mux  Inputs=3
  deuler/dt : Outport
  wires:
  Mux1/1 -> deuler/dt/1
  Fcn2/1 -> Mux1/3
  Fcn1/1 -> Mux1/2
  Fcn/1 -> Mux1/1
  Mux/1 -> Fcn2/1, Fcn1/1, Fcn/1
  euler/1 -> Mux/2
  omega/1 -> Mux/1

== system aero_sim_lib/omega_to_euler/Body-based-to-ref-frame-based ==
  note: dF/dt = P + Q sinF tanQ + R cosF tanQ
      | dQ/dt = Q cosF - R sinF
      | dY/dt = Q sinF secQ + R cosF secQ
  omega : Inport  OutDataType=sfix(16)  OutScaling=2^0
  euler : Inport  Port=2  OutDataType=sfix(16)  OutScaling=2^0
  Fcn : Fcn  Expr=u[1]+u[2]*sin(u[4])*tan(u[5])+u[3]*cos(u[4])*tan(u[5])
  Fcn1 : Fcn  Expr=u[2]*cos(u[4])-u[3]*sin(u[4])
  Fcn2 : Fcn  Expr=u[2]*(sin(u[4])/cos(u[5])) + u[3]*(cos(u[4])/cos(u[5]))
  Mux : Mux  Inputs=2
  Mux1 : Mux  Inputs=3
  deuler/dt : Outport  OutDataType=sfix(16)  OutScaling=2^0
  wires:
  omega/1 -> Mux/1
  euler/1 -> Mux/2
  Mux/1 -> Fcn/1, Fcn1/1, Fcn2/1
  Fcn/1 -> Mux1/1
  Fcn1/1 -> Mux1/2
  Fcn2/1 -> Mux1/3
  Mux1/1 -> deuler/dt/1

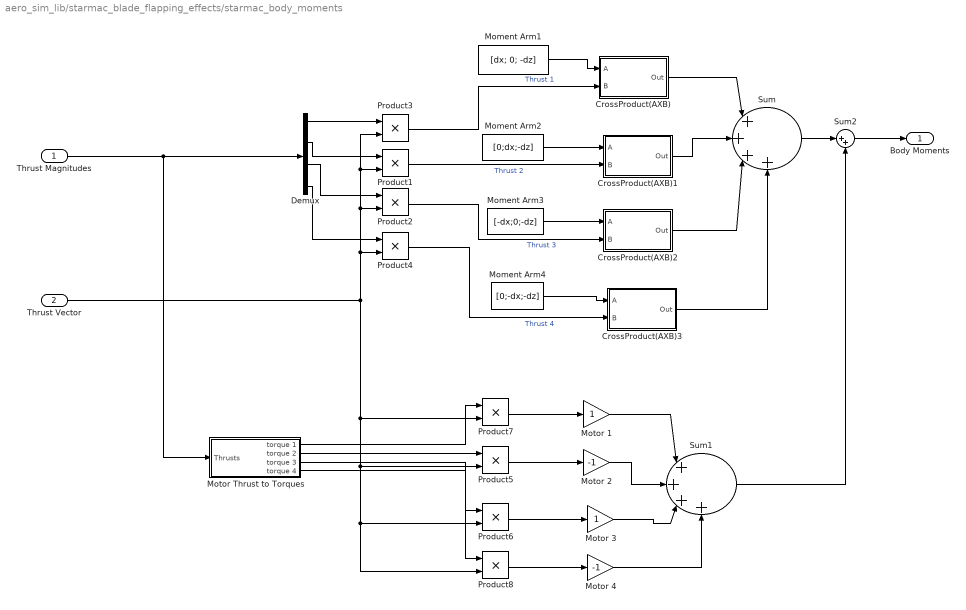
== system aero_sim_lib/starmac_blade_flapping_effects/starmac_body_moments ==
  Thrust Magnitudes : Inport  OutDataType=sfix(16)  OutScaling=2^0
  Thrust Vector : Inport  Port=2  OutDataType=sfix(16)  OutScaling=2^0
  CrossProduct(AXB) : Subsystem
  CrossProduct(AXB)1 : Subsystem
  CrossProduct(AXB)2 : Subsystem
  CrossProduct(AXB)3 : Subsystem
  Demux : Demux
  Moment Arm1 : Constant  Value=[dx; 0; -dz]  OutDataType=sfix(16)  OutScaling=2^0
  Moment Arm2 : Constant  Value=[0;dx;-dz]  OutDataType=sfix(16)  OutScaling=2^0
  Moment Arm3 : Constant  Value=[-dx;0;-dz]  OutDataType=sfix(16)  OutScaling=2^0
  Moment Arm4 : Constant  Value=[0;-dx;-dz]  OutDataType=sfix(16)  OutScaling=2^0
  Motor 1 : Gain  ParameterDataType=sfix(16)  ParameterScaling=2^0  OutDataType=sfix(16)  OutScaling=2^0
  Motor 2 : Gain  Gain=-1  ParameterDataType=sfix(16)  ParameterScaling=2^0  OutDataType=sfix(16)  OutScaling=2^0
  Motor 3 : Gain  ParameterDataType=sfix(16)  ParameterScaling=2^0  OutDataType=sfix(16)  OutScaling=2^0
  Motor 4 : Gain  Gain=-1  ParameterDataType=sfix(16)  ParameterScaling=2^0  OutDataType=sfix(16)  OutScaling=2^0
  Motor Thrust to Torques : Subsystem
  Product{1..8} (8 alike) : Product  OutDataType=sfix(16)  OutScaling=2^0  RndMeth=Zero
  Sum : Sum  Inputs=|++++  OutDataType=sfix(16)  OutScaling=2^0
  Sum1 : Sum  Inputs=|++++  OutDataType=sfix(16)  OutScaling=2^0
  Sum2 : Sum  Inputs=|++  OutDataType=sfix(16)  OutScaling=2^0
  Body Moments : Outport  OutDataType=sfix(16)  OutScaling=2^0
  wires:
  Thrust Magnitudes/1 -> Demux/1, Motor Thrust to Torques/1(Thrusts)
  Demux/1 -> Product3/1
  Demux/2 -> Product1/1
  Demux/3 -> Product2/1
  Demux/4 -> Product4/1
  Thrust Vector/1 -> Product3/2, Product1/2, Product2/2, Product4/2, Product7/2, Product5/2, Product6/2, Product8/2
  Moment Arm1/1 -> CrossProduct(AXB)/1(A)
  Product3/1 -> CrossProduct(AXB)/2(B)  "Thrust 1"
  Moment Arm2/1 -> CrossProduct(AXB)1/1(A)
  Product1/1 -> CrossProduct(AXB)1/2(B)  "Thrust 2"
  Moment Arm3/1 -> CrossProduct(AXB)2/1(A)
  Product2/1 -> CrossProduct(AXB)2/2(B)  "Thrust 3"
  Moment Arm4/1 -> CrossProduct(AXB)3/1(A)
  Product4/1 -> CrossProduct(AXB)3/2(B)  "Thrust 4"
  CrossProduct(AXB)/1(Out) -> Sum/1
  CrossProduct(AXB)2/1(Out) -> Sum/3
  CrossProduct(AXB)3/1(Out) -> Sum/4
  Motor 1/1 -> Sum1/1
  Motor 2/1 -> Sum1/2
  Motor 3/1 -> Sum1/3
  Motor 4/1 -> Sum1/4
  Sum/1 -> Sum2/1
  Sum1/1 -> Sum2/2
  Sum2/1 -> Body Moments/1
  Product7/1 -> Motor 1/1
  Product5/1 -> Motor 2/1
  Product6/1 -> Motor 3/1
  Product8/1 -> Motor 4/1
  Motor Thrust to Torques/1(torque 1) -> Product7/1
  Motor Thrust to Torques/2(torque 2) -> Product5/1
  Motor Thrust to Torques/3(torque 3) -> Product6/1
  Motor Thrust to Torques/4(torque 4) -> Product8/1
  CrossProduct(AXB)1/1(Out) -> Sum/2

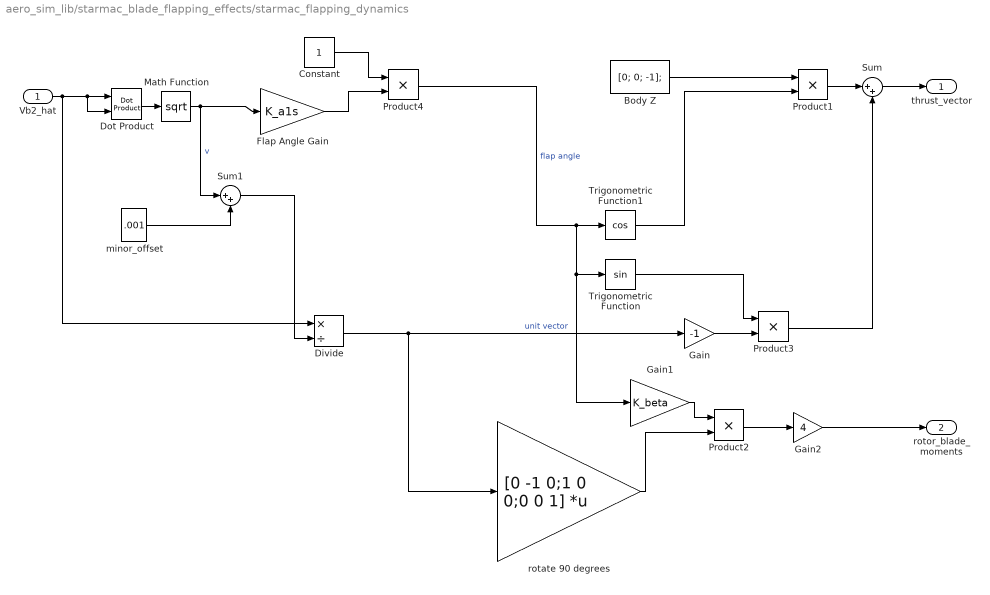
== system aero_sim_lib/starmac_blade_flapping_effects/starmac_flapping_dynamics ==
  Vb2_hat : Inport  OutDataType=sfix(16)  OutScaling=2^0
  "Body Z " : Constant  Value=[0; 0; -1];  OutDataType=sfix(16)  OutScaling=2^0
  Constant : Constant  OutDataType=sfix(16)  OutScaling=2^0
  Divide : Product  Inputs=*/  OutDataType=sfix(16)  OutScaling=2^-10
  Dot Product : simulink/Math Operations/Dot Product  InputSameDT=on  OutDataType=sfix(16)  OutScaling=2^-10  DoSatur=off
  Flap Angle Gain : Gain  Gain=K_a1s  ParameterDataType=sfix(16)  ParameterScaling=2^0  OutDataType=sfix(16)  OutScaling=2^0
  Gain : Gain  Gain=-1  ParameterDataType=sfix(16)  ParameterScaling=2^0  OutDataType=sfix(16)  OutScaling=2^0
  Gain1 : Gain  Gain=K_beta  ParameterDataType=sfix(16)  ParameterScaling=2^0  OutDataType=sfix(16)  OutScaling=2^0
  Gain2 : Gain  Gain=4  ParameterDataType=sfix(16)  ParameterScaling=2^0  OutDataType=sfix(16)  OutScaling=2^0
  Math Function : Math  Operator=sqrt  OutDataType=sfix(16)  OutScaling=2^0  SaturateOnIntegerOverflow=on
  Product{1..4} (4 alike) : Product  OutDataType=sfix(16)  OutScaling=2^0  RndMeth=Zero
  Sum : Sum  Inputs=|++  OutDataType=sfix(16)  OutScaling=2^0
  Sum1 : Sum  Inputs=|++  OutDataType=sfix(16)  OutScaling=2^0
  Trigonometric Function : Trigonometry
  Trigonometric Function1 : Trigonometry  Operator=cos
  minor_offset : Constant  Value=.001  OutDataType=sfix(16)  OutScaling=2^0
  rotate 90 degrees : Gain  Gain=[0 -1 0;1 0 0;0 0 1]  Multiplication=Matrix(K*u)  ParameterDataType=sfix(16)  ParameterScaling=2^0  OutDataType=sfix(16)  OutScaling=2^0
  thrust_vector : Outport  OutDataType=sfix(16)  OutScaling=2^0
  rotor_blade_moments : Outport  Port=2  OutDataType=sfix(16)  OutScaling=2^0
  wires:
  Constant/1 -> Product4/1
  Flap Angle Gain/1 -> Product4/2
  Gain1/1 -> Product2/1
  rotate 90 degrees/1 -> Product2/2
  Product2/1 -> Gain2/1
  Gain2/1 -> rotor_blade_moments/1
  Sum/1 -> thrust_vector/1
  "Body Z "/1 -> Product1/1
  Product1/1 -> Sum/1
  Gain/1 -> Product3/2
  Product3/1 -> Sum/2
  Trigonometric Function/1 -> Product3/1
  Trigonometric Function1/1 -> Product1/2
  Math Function/1 -> Flap Angle Gain/1, Sum1/1  "v"
  Dot Product/1 -> Math Function/1
  Vb2_hat/1 -> Dot Product/2, Dot Product/1, Divide/1
  Product4/1 -> Gain1/1, Trigonometric Function/1, Trigonometric Function1/1  "flap angle"
  Divide/1 -> Gain/1, rotate 90 degrees/1  "unit vector"
  Sum1/1 -> Divide/2
  minor_offset/1 -> Sum1/2

== system aero_sim_lib/starmac_blade_flapping_effects/starmac_vertical_effect_dynamics ==
  motor_thrusts : Inport  OutDataType=sfix(16)  OutScaling=2^0
  v_body_relative : Inport  Port=2  OutDataType=sfix(16)  OutScaling=2^0
  Demux : Demux
  Mux : Mux
  starmac_motor_vertical_effect_dynamics{,1..3} (4 alike) : aero_sim_lib/starmac_motor_vertical_effect_dynamics  SystemSampleTime=-1  tau_motor=tau_motor  R=R  Alpha=Alpha  Vinf=Vinf  Vh=Vh  ToverTh=ToverTh
  thrust_multiplier : Outport  OutDataType=sfix(16)  OutScaling=2^0
  wires:
  v_body_relative/1 -> starmac_motor_vertical_effect_dynamics/2, starmac_motor_vertical_effect_dynamics1/2, starmac_motor_vertical_effect_dynamics3/2, starmac_motor_vertical_effect_dynamics2/2
  starmac_motor_vertical_effect_dynamics3/1 -> Mux/4
  starmac_motor_vertical_effect_dynamics2/1 -> Mux/3
  starmac_motor_vertical_effect_dynamics1/1 -> Mux/2
  starmac_motor_vertical_effect_dynamics/1 -> Mux/1
  Demux/4 -> starmac_motor_vertical_effect_dynamics3/1
  Demux/3 -> starmac_motor_vertical_effect_dynamics2/1
  Demux/2 -> starmac_motor_vertical_effect_dynamics1/1
  Demux/1 -> starmac_motor_vertical_effect_dynamics/1
  Mux/1 -> thrust_multiplier/1
  motor_thrusts/1 -> Demux/1

== system aero_sim_lib/starmac_body_moments/CrossProduct(AXB) ==
  A : Inport  OutDataType=sfix(16)  OutScaling=2^0
  B : Inport  Port=2  OutDataType=sfix(16)  OutScaling=2^0
  Fcn : Fcn  Expr=u[2]*u[6]-u[3]*u[5]
  Fcn1 : Fcn  Expr=u[3]*u[4]-u[1]*u[6]
  Fcn2 : Fcn  Expr=u[1]*u[5]-u[2]*u[4]
  Mux : Mux  Inputs=2
  Mux1 : Mux  Inputs=3
  Out : Outport  OutDataType=sfix(16)  OutScaling=2^0
  wires:
  Mux1/1 -> Out/1
  Fcn2/1 -> Mux1/3
  Fcn1/1 -> Mux1/2
  Fcn/1 -> Mux1/1
  Mux/1 -> Fcn2/1, Fcn1/1, Fcn/1
  B/1 -> Mux/2
  A/1 -> Mux/1
